simulink model "matcher_simu"  (R2019b)
settings: Solver=FixedStepDiscrete  StartTime=0.0  StopTime=N_sym  RelTol=1e-3
InitFcn:
  | %% DSPBuilder Start
  | alt_dspbuilder_update_model(bdroot)
  | %% DSPBuilder End
  | 
  | matcher_init
StartFcn:
  | %% DSPBuilder Start
  | alt_dspbuilder_hdlimport_prepare_for_simulation(bdroot)
  | %% DSPBuilder End
StopFcn:
  | matcher_analysis
libraries: dspsrcs4 x4
settings Model: Creator=vboxuser  LastModifiedBy=vboxuser
settings DataIOCC: SaveFormat=Array

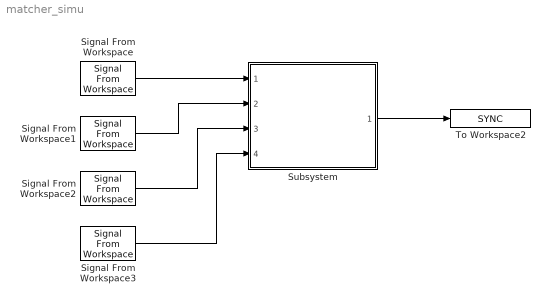
== system matcher_simu ==
  Signal From Workspace : dspsrcs4/Signal From Workspace  X=matcher_match  Ts=1  nsamps=1  OutputAfterFinalValue=Setting to zero  ignoreOrWarnInputAndFrameLengths=off  OutputFrames=off
  Signal From Workspace1 : dspsrcs4/Signal From Workspace  X=matcher_valid  Ts=1  nsamps=1  OutputAfterFinalValue=Setting to zero  ignoreOrWarnInputAndFrameLengths=off  OutputFrames=off
  Signal From Workspace2 : dspsrcs4/Signal From Workspace  X=matcher_en  Ts=1  nsamps=1  OutputAfterFinalValue=Setting to zero  ignoreOrWarnInputAndFrameLengths=off  OutputFrames=off
  Signal From Workspace3 : dspsrcs4/Signal From Workspace  X=matcher_reset  Ts=1  nsamps=1  OutputAfterFinalValue=Setting to zero  ignoreOrWarnInputAndFrameLengths=off  OutputFrames=off
  Subsystem : Subsystem  ReferencedSubsystem=matcher
  To Workspace2 : ToWorkspace  VariableName=SYNC  SampleTime=-1
      settings: Save2DSignal=2-D array (concatenate along first dimension)
  wires:
  Signal From Workspace/1 -> Subsystem/1
  Signal From Workspace1/1 -> Subsystem/2
  Signal From Workspace2/1 -> Subsystem/3
  Signal From Workspace3/1 -> Subsystem/4
  Subsystem/1 -> To Workspace2/1
